simulink model "VOO_proof_of_concept"  (R2020a)
settings: Solver=FixedStepAuto  StartTime=0.0  StopTime=10.0  FixedStep=1e-3  RelTol=1e-3  EnableMultiTasking=on
model workspace (MAT data in the model file):
  ATR_CMP_REF_PWM_PERCENTAGE = 50
  PACING_REF_PWM_DUTY_PERCENTAGE = 50
  VENT_CMP_REF_PWM_PERCENTAGE = 50
settings Model: ExtModeTrigDuration=5  OrderedModelArguments=off  Creator=John  LastModifiedBy=Ethan
settings OptimizationCC: EnhancedBackFolding=on  PassReuseOutputArgsAs=Individual arguments  ZeroExternalMemoryAtStartup=off  ZeroInternalMemoryAtStartup=off  MaxStackSize=64  OptimizeBlockOrder=speed  DifferentSizesBufferReuse=on  OptimizationCustomize=off  EfficientTunableParamExpr=on
settings DebuggingCC: ParameterTunabilityLossMsg=error
settings HardwareCC: ProdBitPerPointer=32  ProdBitPerSizeT=32  ProdBitPerPtrDiffT=32  ProdLargestAtomicInteger=Long  ProdLargestAtomicFloat=Double  ProdWordSize=32  ProdHWDeviceType=ARM Compatible->ARM Cortex
settings SFSimCC: MATLABDynamicMemAlloc=off
settings RTWCC: SystemTargetFile=ert.tlc  HardwareBoard=NXP FRDM-K64F  TemplateMakefile=ert_default_tmf  Toolchain=GNU Tools for ARM Embedded Processors
settings CodeAppCC: ForceParamTrailComments=on  IgnoreCustomStorageClasses=off  OperatorAnnotations=on  SimulinkDataObjDesc=on  SFDataObjDesc=on  InsertBlockDesc=on

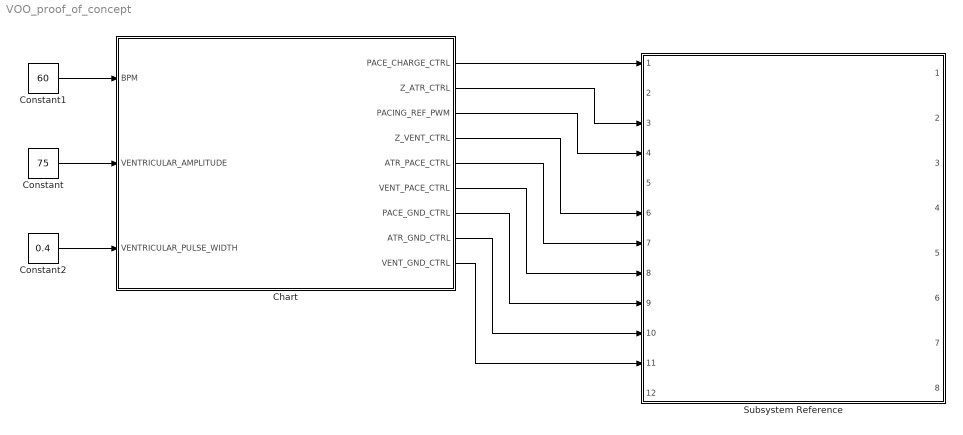
== system VOO_proof_of_concept ==
  Chart : Stateflow chart  TreatAsAtomicUnit=on
      settings: PortSchema="{\"entries\":[{\"content\":{\"sides\":[{\"content\":{\"connectorIds\":[\"In1\",\"In2\",\"In3\"]},\"type\":\"ConnectorPlacement.EquallySpacedRectSide\",\"uuid\":\"a22e05d8-b46e-41db-a99f-a3bab389e16c\"},{\"content\":{\"connectorIds\":[\"Out3\",\"Out8\",\"Out5\",\"Out9\",\"Out2\",\"Out7\",\"Out4\",\"Out1\",\"Out6\"],\"side\":\"RIGHT\"},\"type\":\"ConnectorPlacement.EquallySpacedRectSide\",\"uuid\":\"b830ec1d-656a-4b92-afcd-8fda6b31ad8a\"},{\"content\":{\"connectorIds\":[],\"side\":\"TOP\"},\"type\":\"ConnectorPlacement.EquallySpacedRectSide\",\"uuid\":\"956e5d71-b4a8-48ca-aae1-84adff4c1ec1\"}]},\"type\":\"ConnectorPlacement.EquallySpacedConnector\",\"uuid\":\"bd48be11-38ec-46b0-b71c-a53820608697\"}],\"packageUris\":[\"http://schema.mathworks.com/mf0/Connector/19700101\"],\"version\":\"1.0\"}"
  Constant : Constant  Value=75
  Constant1 : Constant  Value=60
  Constant2 : Constant  Value=0.4
  Subsystem Reference : Subsystem  ReferencedSubsystem=k64f_subsystem
  wires:
  Chart/1(ATR_GND_CTRL) -> Subsystem Reference/10
  Chart/2(ATR_PACE_CTRL) -> Subsystem Reference/7
  Chart/3(PACE_CHARGE_CTRL) -> Subsystem Reference/1
  Chart/4(PACE_GND_CTRL) -> Subsystem Reference/9
  Chart/5(PACING_REF_PWM) -> Subsystem Reference/4
  Chart/6(VENT_GND_CTRL) -> Subsystem Reference/11
  Chart/7(VENT_PACE_CTRL) -> Subsystem Reference/8
  Chart/8(Z_ATR_CTRL) -> Subsystem Reference/3
  Chart/9(Z_VENT_CTRL) -> Subsystem Reference/6
  Constant1/1 -> Chart/1(BPM)
  Constant/1 -> Chart/2(VENTRICULAR_AMPLITUDE)
  Constant2/1 -> Chart/3(VENTRICULAR_PULSE_WIDTH)

== stateflow chart VOO_proof_of_concept/Chart ==
  state PULSE_VENT
    entry:
    PACE_CHARGE_CTRL = 0;
    PACE_GND_CTRL = 1;
    ATR_PACE_CTRL = 0;
    ATR_GND_CTRL = 0;
    Z_ATR_CTRL = 0;
    Z_VENT_CTRL = 0;
    VENT_GND_CTRL = 0;
    VENT_PACE_CTRL = 1;
  state CHARGE
    entry:
    ATR_PACE_CTRL = 0;
    VENT_PACE_CTRL = 0;
    PACING_REF_PWM = VENTRICULAR_AMPLITUDE;
    PACE_CHARGE_CTRL = 1;
  state DISCHARGE
    entry:
    PACE_GND_CTRL = 1;
    VENT_PACE_CTRL = 0;
    Z_ATR_CTRL = 0;
    Z_VENT_CTRL = 0;
    ATR_PACE_CTRL = 0;
    ATR_GND_CTRL = 0;
    VENT_GND_CTRL = 1;
  (default) -> CHARGE
  CHARGE -> PULSE_VENT : after(60/BPM,sec)
  DISCHARGE -> CHARGE
  PULSE_VENT -> DISCHARGE : after(VENTRICULAR_PULSE_WIDTH, msec)
  data: ATR_GND_CTRL output; ATR_PACE_CTRL output; PACE_CHARGE_CTRL output; PACE_GND_CTRL output; PACING_REF_PWM output; VENT_GND_CTRL output; VENT_PACE_CTRL output; Z_ATR_CTRL output; Z_VENT_CTRL output; BPM input; VENTRICULAR_AMPLITUDE input; VENTRICULAR_PULSE_WIDTH input
